simulink model "admire_linear_test_lin_cs"  (Simulink 3.00)
settings: Solver=ode4  StartTime=0.0  StopTime=30  FixedStep=0.008  RelTol=1e-3
undefined symbols (not defined in the file or in its folder): Abare, Afcs_cs, Bbare, Bfcs_cs, Cbare, Cfcs_cs, Dbare, ddc_bw, ddc_rate, ddei_bw, ddei_rate, ddey_bw, ddey_rate, ddle_bw, ddle_rate, ddr_bw, ddr_rate, Dfcs_cs, Mach, rlimit_c, rlimit_ie, rlimit_le, rlimit_oe, rlimit_r, y0bare
libraries: simulink_extras x16
settings Model: TimeSaveName=tout_lin  OutputSaveName=yout_lin  LastModifiedBy=hkg

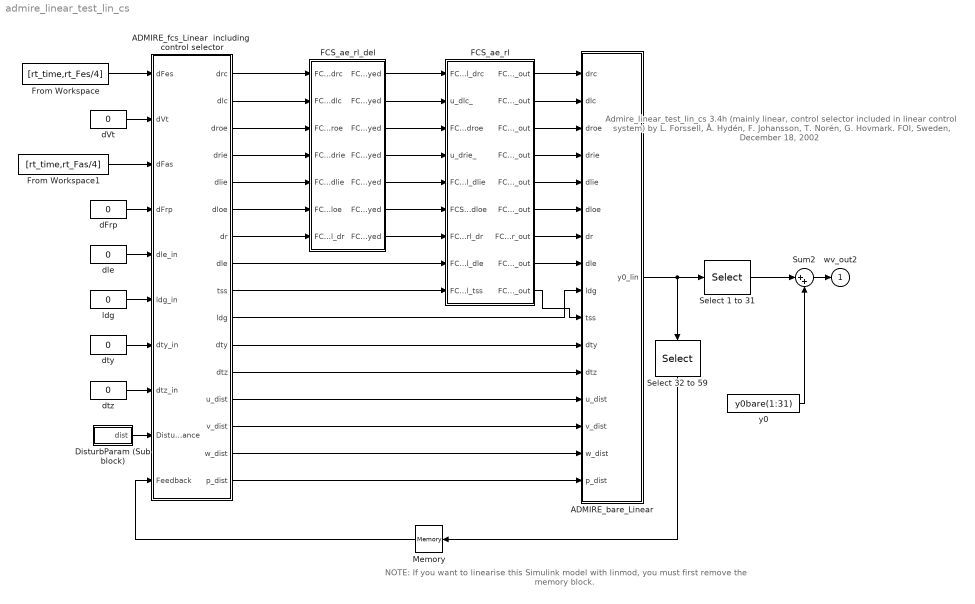
== system admire_linear_test_lin_cs ==
  note: Admire_linear_test_lin_cs 3.4h
      | (mainly linear, control selector included
      | in linear control system)
      | by  L. Forssell,
      | Å. Hydén,
      | F. Johansson,
      | T. Norén,
      | G. Hovmark.
      | FOI, Sweden,
      | December 18, 2002
  note: NOTE: If you want to linearise this Simulink model
      | with linmod, you must first
      | remove the memory block.
  ADMIRE_bare_Linear : Subsystem
  ADMIRE_fcs_Linear  including  control selector : Subsystem
  DisturbParam (Sub block) : Subsystem
  FCS_ae_rl : Subsystem
      mask Display: disp('Saturators,\nRatelimiters\nand\nActuators\n\nMach No and\nrate limiter\ndata are\ntaken from\nWorkspace\n\nAll inital\nstates empty')
  FCS_ae_rl_del : Subsystem
      mask Display: disp('Total\nComputer\nDelay\n\nAll inital\nstates empty')
  From Workspace : FromWorkspace  VariableName=[rt_time,rt_Fes/4]  SampleTime=0  HoldFinalValue=off
  From Workspace1 : FromWorkspace  VariableName=[rt_time,rt_Fas/4]  SampleTime=0  HoldFinalValue=off
  Memory : Memory  Orientation=left  X0=0  InheritSampleTime=off
  Select 1 to 31 : Selector  Elements=[1:31]  InputPortWidth=59
  Select 32 to 59 : Selector  Orientation=down  Elements=[32:59]  InputPortWidth=59
  Sum2 : Sum  Inputs=|++  SaturateOnIntegerOverflow=on
  dFrp : Constant  Value=0
  dVt : Constant  Value=0
  dle : Constant  Value=0
  dty : Constant  Value=0
  dtz : Constant  Value=0
  ldg : Constant  Value=0
  y0 : Constant  Value=y0bare(1:31)
  wv_out2 : Outport  Port=1  InitialOutput=0
  wires:
  ADMIRE_fcs_Linear  including  control selector/16(p_dist) -> ADMIRE_bare_Linear/16(p_dist)
  ADMIRE_fcs_Linear  including  control selector/12(dtz) -> ADMIRE_bare_Linear/12(dtz)
  ADMIRE_fcs_Linear  including  control selector/11(dty) -> ADMIRE_bare_Linear/11(dty)
  FCS_ae_rl_del/1(FCS_ae_rl_del_drc_delayed) -> FCS_ae_rl/1(FCS_ae_rl_drc)
  FCS_ae_rl_del/2(FCS_ae_rl_del_dlc_delayed) -> FCS_ae_rl/2(u_dlc_)
  FCS_ae_rl_del/3(FCS_ae_rl_del_droe_delayed) -> FCS_ae_rl/3(FCS_ae_rl_droe)
  FCS_ae_rl_del/4(FCS_ae_rl_del_drie_delayed) -> FCS_ae_rl/4(u_drie_)
  FCS_ae_rl_del/5(FCS_ae_rl_del_dlie_delayed) -> FCS_ae_rl/5(FCS_ae_rl_dlie)
  FCS_ae_rl_del/6(FCS_ae_rl_del_dloe_delayed) -> FCS_ae_rl/6(FCS_ae_rl_dloe)
  FCS_ae_rl_del/7(FCS_ae_rl_del_dr_delayed) -> FCS_ae_rl/7(FCS_ae_rl_dr)
  ADMIRE_fcs_Linear  including  control selector/8(dle) -> FCS_ae_rl/8(FCS_ae_rl_dle)
  ADMIRE_fcs_Linear  including  control selector/9(tss) -> FCS_ae_rl/9(FCS_ae_rl_tss)
  ADMIRE_fcs_Linear  including  control selector/10(ldg) -> ADMIRE_bare_Linear/9(ldg)
  ADMIRE_fcs_Linear  including  control selector/13(u_dist) -> ADMIRE_bare_Linear/13(u_dist)
  ADMIRE_fcs_Linear  including  control selector/14(v_dist) -> ADMIRE_bare_Linear/14(v_dist)
  ADMIRE_fcs_Linear  including  control selector/15(w_dist) -> ADMIRE_bare_Linear/15(w_dist)
  FCS_ae_rl/1(FCS_ae_rl_drc_out) -> ADMIRE_bare_Linear/1(drc)
  FCS_ae_rl/2(FCS_ae_rl_dlc_out) -> ADMIRE_bare_Linear/2(dlc)
  FCS_ae_rl/3(FCS_ae_rl_droe_out) -> ADMIRE_bare_Linear/3(droe)
  FCS_ae_rl/4(FCS_ae_rl_drie_out) -> ADMIRE_bare_Linear/4(drie)
  FCS_ae_rl/5(FCS_ae_rl_dlie_out) -> ADMIRE_bare_Linear/5(dlie)
  FCS_ae_rl/6(FCS_ae_rl_dloe_out) -> ADMIRE_bare_Linear/6(dloe)
  FCS_ae_rl/7(FCS_ae_rl_dr_out) -> ADMIRE_bare_Linear/7(dr)
  FCS_ae_rl/8(FCS_ae_rl_dle_out) -> ADMIRE_bare_Linear/8(dle)
  FCS_ae_rl/9(FCS_ae_rl_tss_out) -> ADMIRE_bare_Linear/10(tss)
  ADMIRE_bare_Linear/1(y0_lin) -> Select 1 to 31/1, Select 32 to 59/1
  Select 32 to 59/1 -> Memory/1
  Sum2/1 -> wv_out2/1
  y0/1 -> Sum2/2
  Select 1 to 31/1 -> Sum2/1
  Memory/1 -> ADMIRE_fcs_Linear  including  control selector/10(Feedback)
  ADMIRE_fcs_Linear  including  control selector/1(drc) -> FCS_ae_rl_del/1(FCS_ae_rl_del_drc)
  ADMIRE_fcs_Linear  including  control selector/2(dlc) -> FCS_ae_rl_del/2(FCS_ae_rl_del_dlc)
  ADMIRE_fcs_Linear  including  control selector/3(droe) -> FCS_ae_rl_del/3(FCS_ae_rl_del_droe)
  ADMIRE_fcs_Linear  including  control selector/4(drie) -> FCS_ae_rl_del/4(FCS_ae_rl_del_drie)
  ADMIRE_fcs_Linear  including  control selector/5(dlie) -> FCS_ae_rl_del/5(FCS_ae_rl_del_dlie)
  ADMIRE_fcs_Linear  including  control selector/6(dloe) -> FCS_ae_rl_del/6(FCS_ae_rl_del_dloe)
  ADMIRE_fcs_Linear  including  control selector/7(dr) -> FCS_ae_rl_del/7(FCS_ae_rl_del_dr)
  From Workspace/1 -> ADMIRE_fcs_Linear  including  control selector/1(dFes)
  dVt/1 -> ADMIRE_fcs_Linear  including  control selector/2(dVt)
  From Workspace1/1 -> ADMIRE_fcs_Linear  including  control selector/3(dFas)
  dFrp/1 -> ADMIRE_fcs_Linear  including  control selector/4(dFrp)
  dle/1 -> ADMIRE_fcs_Linear  including  control selector/5(dle_in)
  ldg/1 -> ADMIRE_fcs_Linear  including  control selector/6(ldg_in)
  dty/1 -> ADMIRE_fcs_Linear  including  control selector/7(dty_in)
  dtz/1 -> ADMIRE_fcs_Linear  including  control selector/8(dtz_in)
  DisturbParam (Sub block)/1(dist) -> ADMIRE_fcs_Linear  including  control selector/9(Disturbance)

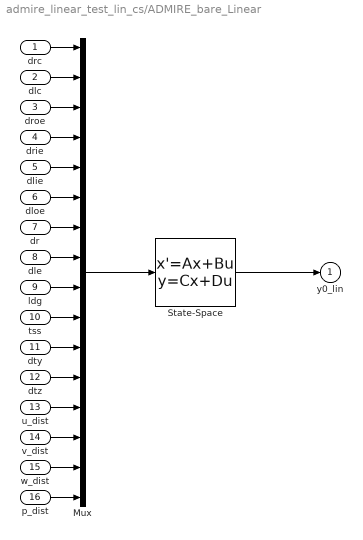
== system admire_linear_test_lin_cs/ADMIRE_bare_Linear ==
  drc : Inport  Port=1  PortWidth=-1  SampleTime=-1  DataType=auto
      settings: SignalType=auto
  dlc : Inport  Port=2  PortWidth=-1  SampleTime=-1  DataType=auto
      settings: SignalType=auto
  droe : Inport  Port=3  PortWidth=-1  SampleTime=-1  DataType=auto
      settings: SignalType=auto
  drie : Inport  Port=4  PortWidth=-1  SampleTime=-1  DataType=auto
      settings: SignalType=auto
  dlie : Inport  Port=5  PortWidth=-1  SampleTime=-1  DataType=auto
      settings: SignalType=auto
  dloe : Inport  Port=6  PortWidth=-1  SampleTime=-1  DataType=auto
      settings: SignalType=auto
  dr : Inport  Port=7  PortWidth=-1  SampleTime=-1  DataType=auto
      settings: SignalType=auto
  dle : Inport  Port=8  PortWidth=-1  SampleTime=-1  DataType=auto
      settings: SignalType=auto
  ldg : Inport  Port=9  PortWidth=-1  SampleTime=-1  DataType=auto
      settings: SignalType=auto
  tss : Inport  Port=10  PortWidth=-1  SampleTime=-1  DataType=auto
      settings: SignalType=auto
  dty : Inport  Port=11  PortWidth=-1  SampleTime=-1  DataType=auto
      settings: SignalType=auto
  dtz : Inport  Port=12  PortWidth=-1  SampleTime=-1  DataType=auto
      settings: SignalType=auto
  u_dist : Inport  Port=13  PortWidth=-1  SampleTime=-1  DataType=auto
      settings: SignalType=auto
  v_dist : Inport  Port=14  PortWidth=-1  SampleTime=-1  DataType=auto
      settings: SignalType=auto
  w_dist : Inport  Port=15  PortWidth=-1  SampleTime=-1  DataType=auto
      settings: SignalType=auto
  p_dist : Inport  Port=16  PortWidth=-1  SampleTime=-1  DataType=auto
      settings: SignalType=auto
  Mux : Mux  Inputs=16
      settings: DisplayOption=none
  State-Space : StateSpace  A=Abare  B=Bbare  C=Cbare  D=Dbare  X0=[]
  y0_lin : Outport  Port=1  InitialOutput=0
  wires:
  w_dist/1 -> Mux/15
  p_dist/1 -> Mux/16
  drc/1 -> Mux/1
  dlc/1 -> Mux/2
  droe/1 -> Mux/3
  drie/1 -> Mux/4
  dlie/1 -> Mux/5
  dloe/1 -> Mux/6
  dr/1 -> Mux/7
  dle/1 -> Mux/8
  ldg/1 -> Mux/9
  tss/1 -> Mux/10
  dty/1 -> Mux/11
  dtz/1 -> Mux/12
  u_dist/1 -> Mux/13
  v_dist/1 -> Mux/14
  Mux/1 -> State-Space/1
  State-Space/1 -> y0_lin/1

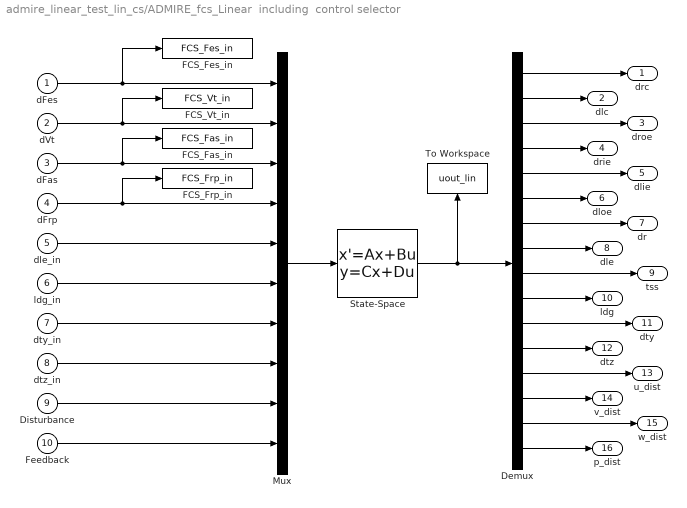
== system admire_linear_test_lin_cs/ADMIRE_fcs_Linear  including  control selector ==
  dFes : Inport  Port=1  PortWidth=-1  SampleTime=-1  DataType=auto
      settings: SignalType=auto
  dVt : Inport  Port=2  PortWidth=-1  SampleTime=-1  DataType=auto
      settings: SignalType=auto
  dFas : Inport  Port=3  PortWidth=-1  SampleTime=-1  DataType=auto
      settings: SignalType=auto
  dFrp : Inport  Port=4  PortWidth=-1  SampleTime=-1  DataType=auto
      settings: SignalType=auto
  dle_in : Inport  Port=5  PortWidth=-1  SampleTime=-1  DataType=auto
      settings: SignalType=auto
  ldg_in : Inport  Port=6  PortWidth=-1  SampleTime=-1  DataType=auto
      settings: SignalType=auto
  dty_in : Inport  Port=7  PortWidth=-1  SampleTime=-1  DataType=auto
      settings: SignalType=auto
  dtz_in : Inport  Port=8  PortWidth=-1  SampleTime=-1  DataType=auto
      settings: SignalType=auto
  Disturbance : Inport  Port=9  PortWidth=-1  SampleTime=-1  DataType=auto
      settings: SignalType=auto
  Feedback : Inport  Port=10  PortWidth=-1  SampleTime=-1  DataType=auto
      settings: SignalType=auto
  Demux : Demux  Outputs=16
  FCS_Fas_in : ToWorkspace  VariableName=FCS_Fas_in  SampleTime=-1  SaveFormat=Matrix
  FCS_Fes_in : ToWorkspace  VariableName=FCS_Fes_in  SampleTime=-1  SaveFormat=Matrix
  FCS_Frp_in : ToWorkspace  VariableName=FCS_Frp_in  SampleTime=-1  SaveFormat=Matrix
  FCS_Vt_in : ToWorkspace  VariableName=FCS_Vt_in  SampleTime=-1  SaveFormat=Matrix
  Mux : Mux  Inputs=10
  State-Space : StateSpace  A=Afcs_cs  B=Bfcs_cs  C=Cfcs_cs  D=Dfcs_cs  X0=[]
  To Workspace : ToWorkspace  VariableName=uout_lin  SampleTime=-1  SaveFormat=Matrix
      settings: Orientation=up
  drc : Outport  Port=1
  dlc : Outport  Port=2
  droe : Outport  Port=3
  drie : Outport  Port=4
  dlie : Outport  Port=5
  dloe : Outport  Port=6
  dr : Outport  Port=7
  dle : Outport  Port=8
  tss : Outport  Port=9
  ldg : Outport  Port=10
  dty : Outport  Port=11
  dtz : Outport  Port=12
  u_dist : Outport  Port=13
  v_dist : Outport  Port=14
  w_dist : Outport  Port=15
  p_dist : Outport  Port=16
  wires:
  Mux/1 -> State-Space/1
  dle_in/1 -> Mux/5
  ldg_in/1 -> Mux/6
  dty_in/1 -> Mux/7
  dtz_in/1 -> Mux/8
  Disturbance/1 -> Mux/9
  Feedback/1 -> Mux/10
  Demux/1 -> drc/1
  Demux/2 -> dlc/1
  Demux/7 -> dr/1
  Demux/8 -> dle/1
  Demux/10 -> ldg/1
  Demux/11 -> dty/1
  Demux/12 -> dtz/1
  Demux/13 -> u_dist/1
  Demux/14 -> v_dist/1
  Demux/15 -> w_dist/1
  Demux/16 -> p_dist/1
  Demux/3 -> droe/1
  Demux/4 -> drie/1
  Demux/5 -> dlie/1
  Demux/6 -> dloe/1
  Demux/9 -> tss/1
  State-Space/1 -> Demux/1, To Workspace/1
  dFes/1 -> Mux/1, FCS_Fes_in/1
  dVt/1 -> Mux/2, FCS_Vt_in/1
  dFrp/1 -> Mux/4, FCS_Frp_in/1
  dFas/1 -> Mux/3, FCS_Fas_in/1

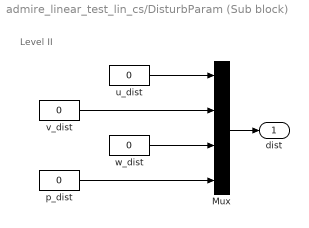
== system admire_linear_test_lin_cs/DisturbParam (Sub block) ==
  note: Level II
  Mux : Mux  Inputs=4
      settings: DisplayOption=none
  "p_dist " : Constant  Value=0
  "u_dist " : Constant  Value=0
  "v_dist " : Constant  Value=0
  "w_dist " : Constant  Value=0
  dist : Outport  Port=1
  wires:
  "p_dist "/1 -> Mux/4
  "w_dist "/1 -> Mux/3
  "v_dist "/1 -> Mux/2
  "u_dist "/1 -> Mux/1
  Mux/1 -> dist/1

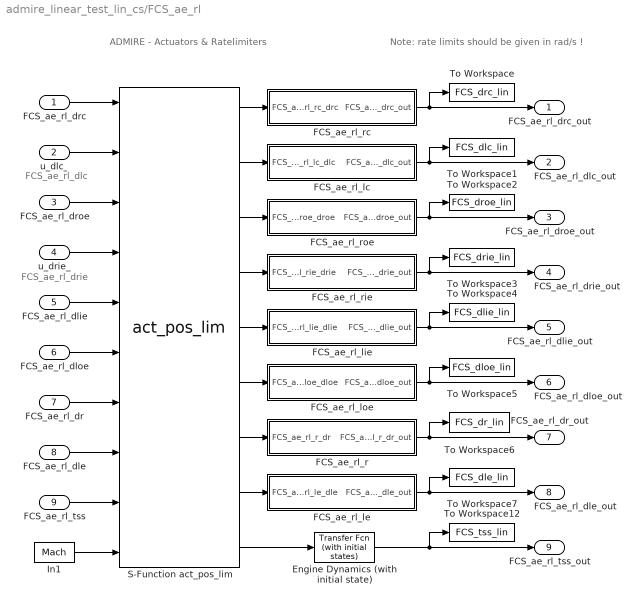
== system admire_linear_test_lin_cs/FCS_ae_rl ==
  note: Note: rate limits should be given
      | in rad/s !
  note: FCS_ae_rl_dlc
  note: FCS_ae_rl_drie
  note: ADMIRE - Actuators & Ratelimiters
  FCS_ae_rl_drc : Inport  Port=1  PortWidth=-1  SampleTime=-1  DataType=auto
      settings: SignalType=auto
  u_dlc_ : Inport  Port=2  PortWidth=-1  SampleTime=-1  DataType=auto
      settings: SignalType=auto
  FCS_ae_rl_droe : Inport  Port=3  PortWidth=-1  SampleTime=-1  DataType=auto
      settings: SignalType=auto
  u_drie_ : Inport  Port=4  PortWidth=-1  SampleTime=-1  DataType=auto
      settings: SignalType=auto
  FCS_ae_rl_dlie : Inport  Port=5  PortWidth=-1  SampleTime=-1  DataType=auto
      settings: SignalType=auto
  FCS_ae_rl_dloe : Inport  Port=6  PortWidth=-1  SampleTime=-1  DataType=auto
      settings: SignalType=auto
  FCS_ae_rl_dr : Inport  Port=7  PortWidth=-1  SampleTime=-1  DataType=auto
      settings: SignalType=auto
  FCS_ae_rl_dle : Inport  Port=8  PortWidth=-1  SampleTime=-1  DataType=auto
      settings: SignalType=auto
  FCS_ae_rl_tss : Inport  Port=9  PortWidth=-1  SampleTime=-1  DataType=auto
      settings: SignalType=auto
  Engine Dynamics (with initial state) : simulink_extras/Additional Linear/Transfer Fcn (with initial states)  N=[1]  D="[2  1]"  X0=[0]
  FCS_ae_rl_lc : Subsystem
      mask Display: disp(' Ratelimiter and Dynamics\nServo: lc')
  FCS_ae_rl_le : Subsystem
      mask Display: disp(' Ratelimiter and Dynamics\nServo: le')
  FCS_ae_rl_lie : Subsystem
      mask Display: disp(' Ratelimiter and Dynamics\nServo: lie')
  FCS_ae_rl_loe : Subsystem
      mask Display: disp(' Ratelimiter and Dynamics\nServo: loe')
  FCS_ae_rl_r : Subsystem
      mask Display: disp(' Ratelimiter and Dynamics\nServo: r')
  FCS_ae_rl_rc : Subsystem
      mask Display: disp(' Ratelimiter and Dynamics\nServo: rc')
  FCS_ae_rl_rie : Subsystem
      mask Display: disp(' Ratelimiter and Dynamics\nServo: rie')
  FCS_ae_rl_roe : Subsystem
      mask Display: disp(' Ratelimiter and Dynamics\nServo: roe')
  In1 : Constant  Value=Mach
  S-Function act_pos_lim : S-Function  FunctionName=act_pos_lim  PortCounts=[]  SFunctionModules=''
      mask Display:
      | plot([-30 30],[-30 30])
      | plot([0 0],[-30 30])
      | plot([-50 50],[0 0])
      | plot([30 50],[30 30])
      | plot([-50 -30],[-30 -30])
      | plot([-5 0],[25 30])
      | plot([5 0],[25 30])
      | plot([45 50],[3 0])
      | plot([45 50],[-3 0])
      | text(-21,26,'out')
      | text(30,-2,'in')
  To Workspace : ToWorkspace  VariableName=FCS_drc_lin  SampleTime=-1  SaveFormat=Matrix
  To Workspace1 : ToWorkspace  VariableName=FCS_dlc_lin  SampleTime=-1  SaveFormat=Matrix
  To Workspace12 : ToWorkspace  VariableName=FCS_tss_lin  SampleTime=-1  SaveFormat=Matrix
  To Workspace2 : ToWorkspace  VariableName=FCS_droe_lin  SampleTime=-1  SaveFormat=Matrix
  To Workspace3 : ToWorkspace  VariableName=FCS_drie_lin  SampleTime=-1  SaveFormat=Matrix
  To Workspace4 : ToWorkspace  VariableName=FCS_dlie_lin  SampleTime=-1  SaveFormat=Matrix
  To Workspace5 : ToWorkspace  VariableName=FCS_dloe_lin  SampleTime=-1  SaveFormat=Matrix
  To Workspace6 : ToWorkspace  VariableName=FCS_dr_lin  SampleTime=-1  SaveFormat=Matrix
  To Workspace7 : ToWorkspace  VariableName=FCS_dle_lin  SampleTime=-1  SaveFormat=Matrix
  FCS_ae_rl_drc_out : Outport  Port=1
  FCS_ae_rl_dlc_out : Outport  Port=2
  FCS_ae_rl_droe_out : Outport  Port=3
  FCS_ae_rl_drie_out : Outport  Port=4
  FCS_ae_rl_dlie_out : Outport  Port=5
  FCS_ae_rl_dloe_out : Outport  Port=6
  FCS_ae_rl_dr_out : Outport  Port=7
  FCS_ae_rl_dle_out : Outport  Port=8
  FCS_ae_rl_tss_out : Outport  Port=9
  wires:
  S-Function act_pos_lim/2 -> FCS_ae_rl_lc/1(FCS_ae_rl_lc_dlc)
  S-Function act_pos_lim/3 -> FCS_ae_rl_roe/1(FCS_ae_rl_roe_droe)
  S-Function act_pos_lim/5 -> FCS_ae_rl_lie/1(FCS_ae_rl_lie_dlie)
  S-Function act_pos_lim/6 -> FCS_ae_rl_loe/1(FCS_ae_rl_loe_dloe)
  S-Function act_pos_lim/7 -> FCS_ae_rl_r/1(FCS_ae_rl_r_dr)
  S-Function act_pos_lim/8 -> FCS_ae_rl_le/1(FCS_ae_rl_le_dle)
  S-Function act_pos_lim/9 -> Engine Dynamics (with initial state)/1
  S-Function act_pos_lim/1 -> FCS_ae_rl_rc/1(FCS_ae_rl_rc_drc)
  S-Function act_pos_lim/4 -> FCS_ae_rl_rie/1(FCS_ae_rl_rie_drie)
  In1/1 -> S-Function act_pos_lim/10
  u_dlc_/1 -> S-Function act_pos_lim/2
  FCS_ae_rl_drc/1 -> S-Function act_pos_lim/1
  FCS_ae_rl_droe/1 -> S-Function act_pos_lim/3
  FCS_ae_rl_dlie/1 -> S-Function act_pos_lim/5
  FCS_ae_rl_dloe/1 -> S-Function act_pos_lim/6
  FCS_ae_rl_dr/1 -> S-Function act_pos_lim/7
  u_drie_/1 -> S-Function act_pos_lim/4
  FCS_ae_rl_dle/1 -> S-Function act_pos_lim/8
  FCS_ae_rl_tss/1 -> S-Function act_pos_lim/9
  FCS_ae_rl_rc/1(FCS_ae_rl_rc_drc_out) -> To Workspace/1, FCS_ae_rl_drc_out/1
  FCS_ae_rl_lc/1(FCS_ae_rl_lc_dlc_out) -> To Workspace1/1, FCS_ae_rl_dlc_out/1
  Engine Dynamics (with initial state)/1 -> To Workspace12/1, FCS_ae_rl_tss_out/1
  FCS_ae_rl_le/1(FCS_ae_rl_le_dle_out) -> To Workspace7/1, FCS_ae_rl_dle_out/1
  FCS_ae_rl_r/1(FCS_ae_rl_r_dr_out) -> To Workspace6/1, FCS_ae_rl_dr_out/1
  FCS_ae_rl_loe/1(FCS_ae_rl_loe_dloe_out) -> To Workspace5/1, FCS_ae_rl_dloe_out/1
  FCS_ae_rl_lie/1(FCS_ae_rl_lie_dlie_out) -> To Workspace4/1, FCS_ae_rl_dlie_out/1
  FCS_ae_rl_roe/1(FCS_ae_rl_roe_droe_out) -> To Workspace2/1, FCS_ae_rl_droe_out/1
  FCS_ae_rl_rie/1(FCS_ae_rl_rie_drie_out) -> To Workspace3/1, FCS_ae_rl_drie_out/1

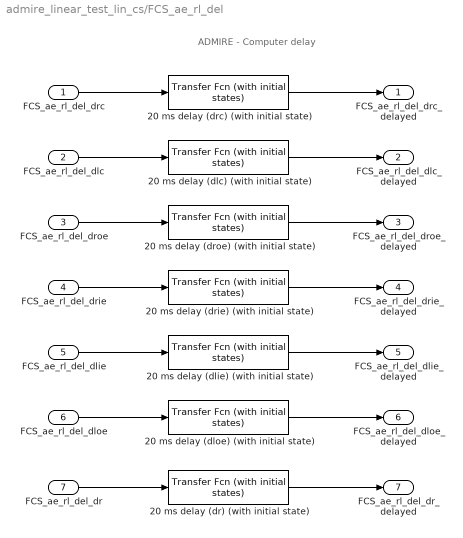
== system admire_linear_test_lin_cs/FCS_ae_rl_del ==
  note: ADMIRE - Computer delay
  FCS_ae_rl_del_drc : Inport  Port=1  PortWidth=-1  SampleTime=-1  DataType=auto
      settings: SignalType=auto
  FCS_ae_rl_del_dlc : Inport  Port=2  PortWidth=-1  SampleTime=-1  DataType=auto
      settings: SignalType=auto
  FCS_ae_rl_del_droe : Inport  Port=3  PortWidth=-1  SampleTime=-1  DataType=auto
      settings: SignalType=auto
  FCS_ae_rl_del_drie : Inport  Port=4  PortWidth=-1  SampleTime=-1  DataType=auto
      settings: SignalType=auto
  FCS_ae_rl_del_dlie : Inport  Port=5  PortWidth=-1  SampleTime=-1  DataType=auto
      settings: SignalType=auto
  FCS_ae_rl_del_dloe : Inport  Port=6  PortWidth=-1  SampleTime=-1  DataType=auto
      settings: SignalType=auto
  FCS_ae_rl_del_dr : Inport  Port=7  PortWidth=-1  SampleTime=-1  DataType=auto
      settings: SignalType=auto
  20 ms delay (dlc) (with initial state) : simulink_extras/Additional Linear/Transfer Fcn (with initial states)  N=[0.000033 -0.01 1]  D=[0.000033 0.01 1]  X0=[]
  20 ms delay (dlie) (with initial state) : simulink_extras/Additional Linear/Transfer Fcn (with initial states)  N=[0.000033 -0.01 1]  D=[0.000033 0.01 1]  X0=[]
  20 ms delay (dloe) (with initial state) : simulink_extras/Additional Linear/Transfer Fcn (with initial states)  N=[0.000033 -0.01 1]  D=[0.000033 0.01 1]  X0=[]
  20 ms delay (dr) (with initial state) : simulink_extras/Additional Linear/Transfer Fcn (with initial states)  N=[0.000033 -0.01 1]  D=[0.000033 0.01 1]  X0=[]
  20 ms delay (drc) (with initial state) : simulink_extras/Additional Linear/Transfer Fcn (with initial states)  N=[0.000033 -0.01 1]  D=[0.000033 0.01 1]  X0=[]
  20 ms delay (drie) (with initial state) : simulink_extras/Additional Linear/Transfer Fcn (with initial states)  N=[0.000033 -0.01 1]  D=[0.000033 0.01 1]  X0=[]
  20 ms delay (droe) (with initial state) : simulink_extras/Additional Linear/Transfer Fcn (with initial states)  N=[0.000033 -0.01 1]  D=[0.000033 0.01 1]  X0=[]
  FCS_ae_rl_del_drc_delayed : Outport  Port=1
  FCS_ae_rl_del_dlc_delayed : Outport  Port=2
  FCS_ae_rl_del_droe_delayed : Outport  Port=3
  FCS_ae_rl_del_drie_delayed : Outport  Port=4
  FCS_ae_rl_del_dlie_delayed : Outport  Port=5
  FCS_ae_rl_del_dloe_delayed : Outport  Port=6
  FCS_ae_rl_del_dr_delayed : Outport  Port=7
  wires:
  FCS_ae_rl_del_drc/1 -> 20 ms delay (drc) (with initial state)/1
  FCS_ae_rl_del_dlc/1 -> 20 ms delay (dlc) (with initial state)/1
  FCS_ae_rl_del_droe/1 -> 20 ms delay (droe) (with initial state)/1
  FCS_ae_rl_del_drie/1 -> 20 ms delay (drie) (with initial state)/1
  FCS_ae_rl_del_dlie/1 -> 20 ms delay (dlie) (with initial state)/1
  FCS_ae_rl_del_dloe/1 -> 20 ms delay (dloe) (with initial state)/1
  FCS_ae_rl_del_dr/1 -> 20 ms delay (dr) (with initial state)/1
  20 ms delay (drc) (with initial state)/1 -> FCS_ae_rl_del_drc_delayed/1
  20 ms delay (dlc) (with initial state)/1 -> FCS_ae_rl_del_dlc_delayed/1
  20 ms delay (droe) (with initial state)/1 -> FCS_ae_rl_del_droe_delayed/1
  20 ms delay (drie) (with initial state)/1 -> FCS_ae_rl_del_drie_delayed/1
  20 ms delay (dlie) (with initial state)/1 -> FCS_ae_rl_del_dlie_delayed/1
  20 ms delay (dloe) (with initial state)/1 -> FCS_ae_rl_del_dloe_delayed/1
  20 ms delay (dr) (with initial state)/1 -> FCS_ae_rl_del_dr_delayed/1

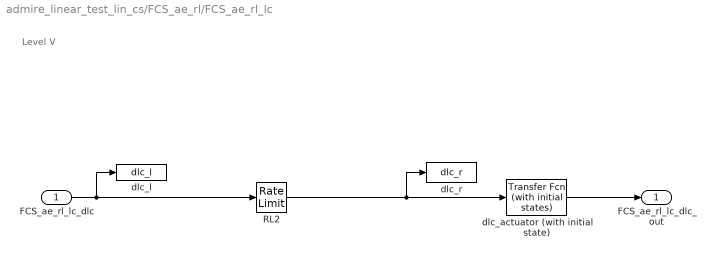
== system admire_linear_test_lin_cs/FCS_ae_rl/FCS_ae_rl_lc ==
  note: Level V
  FCS_ae_rl_lc_dlc : Inport  Port=1  PortWidth=-1  SampleTime=-1  DataType=auto
      settings: SignalType=auto
  RL2 : RateLimiter  RisingSlewLimit=rlimit_c+ddc_rate  FallingSlewLimit=-rlimit_c-ddc_rate
  dlc_actuator (with initial state) : simulink_extras/Additional Linear/Transfer Fcn (with initial states)  N=[1]  D="[0.05+ddc_bw  1]"  X0=[]
  dlc_l : ToWorkspace  VariableName=dlc_l  SampleTime=0  SaveFormat=Matrix
      settings: Buffer=10000
  dlc_r : ToWorkspace  VariableName=dlc_r  SampleTime=0  SaveFormat=Matrix
      settings: Buffer=10000
  FCS_ae_rl_lc_dlc_out : Outport  Port=1  InitialOutput=0
  wires:
  FCS_ae_rl_lc_dlc/1 -> dlc_l/1, RL2/1
  dlc_actuator (with initial state)/1 -> FCS_ae_rl_lc_dlc_out/1
  RL2/1 -> dlc_r/1, dlc_actuator (with initial state)/1

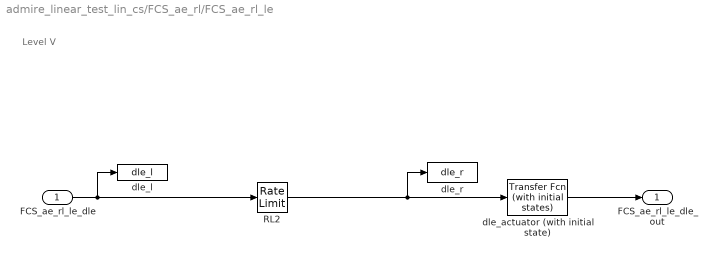
== system admire_linear_test_lin_cs/FCS_ae_rl/FCS_ae_rl_le ==
  note: Level V
  FCS_ae_rl_le_dle : Inport  Port=1  PortWidth=-1  SampleTime=-1  DataType=auto
      settings: SignalType=auto
  RL2 : RateLimiter  RisingSlewLimit=rlimit_le+ddle_rate  FallingSlewLimit=-rlimit_le-ddle_rate
  dle_actuator (with initial state) : simulink_extras/Additional Linear/Transfer Fcn (with initial states)  N=[1]  D="[0.05+ddle_bw  1]"  X0=[0]
  dle_l : ToWorkspace  VariableName=dle_l  SampleTime=0  SaveFormat=Matrix
      settings: Buffer=10000
  dle_r : ToWorkspace  VariableName=dle_r  SampleTime=0  SaveFormat=Matrix
      settings: Buffer=10000
  FCS_ae_rl_le_dle_out : Outport  Port=1  InitialOutput=0
  wires:
  FCS_ae_rl_le_dle/1 -> dle_l/1, RL2/1
  dle_actuator (with initial state)/1 -> FCS_ae_rl_le_dle_out/1
  RL2/1 -> dle_r/1, dle_actuator (with initial state)/1

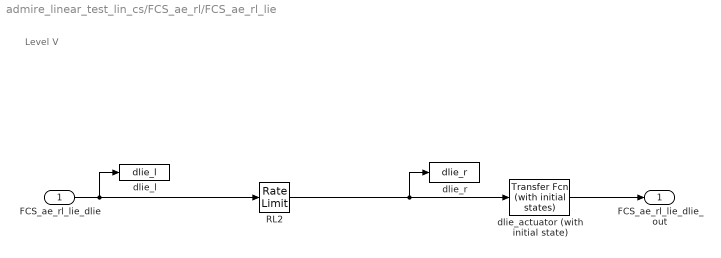
== system admire_linear_test_lin_cs/FCS_ae_rl/FCS_ae_rl_lie ==
  note: Level V
  FCS_ae_rl_lie_dlie : Inport  Port=1  PortWidth=-1  SampleTime=-1  DataType=auto
      settings: SignalType=auto
  RL2 : RateLimiter  RisingSlewLimit=rlimit_ie+ddei_rate  FallingSlewLimit=-rlimit_ie-ddei_rate
  dlie_actuator (with initial state) : simulink_extras/Additional Linear/Transfer Fcn (with initial states)  N=[1]  D="[0.05+ddei_bw  1]"  X0=[0]
  dlie_l : ToWorkspace  VariableName=dlie_l  SampleTime=0  SaveFormat=Matrix
      settings: Buffer=10000
  dlie_r : ToWorkspace  VariableName=dlie_r  SampleTime=0  SaveFormat=Matrix
      settings: Buffer=10000
  FCS_ae_rl_lie_dlie_out : Outport  Port=1  InitialOutput=0
  wires:
  dlie_actuator (with initial state)/1 -> FCS_ae_rl_lie_dlie_out/1
  FCS_ae_rl_lie_dlie/1 -> dlie_l/1, RL2/1
  RL2/1 -> dlie_actuator (with initial state)/1, dlie_r/1

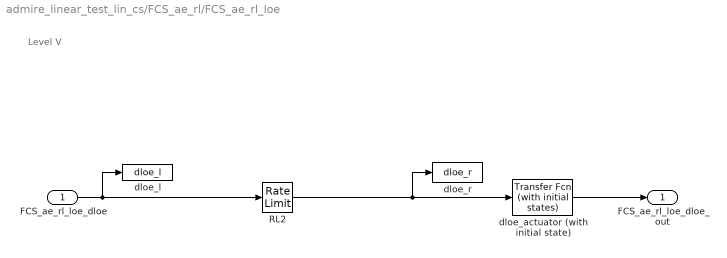
== system admire_linear_test_lin_cs/FCS_ae_rl/FCS_ae_rl_loe ==
  note: Level V
  FCS_ae_rl_loe_dloe : Inport  Port=1  PortWidth=-1  SampleTime=-1  DataType=auto
      settings: SignalType=auto
  RL2 : RateLimiter  RisingSlewLimit=rlimit_oe+ddey_rate  FallingSlewLimit=-rlimit_oe-ddey_rate
  dloe_actuator (with initial state) : simulink_extras/Additional Linear/Transfer Fcn (with initial states)  N=[1]  D="[0.05+ddey_bw  1]"  X0=[0]
  dloe_l : ToWorkspace  VariableName=dloe_l  SampleTime=0  SaveFormat=Matrix
      settings: Buffer=10000
  dloe_r : ToWorkspace  VariableName=dloe_r  SampleTime=0  SaveFormat=Matrix
      settings: Buffer=10000
  FCS_ae_rl_loe_dloe_out : Outport  Port=1  InitialOutput=0
  wires:
  FCS_ae_rl_loe_dloe/1 -> dloe_l/1, RL2/1
  dloe_actuator (with initial state)/1 -> FCS_ae_rl_loe_dloe_out/1
  RL2/1 -> dloe_r/1, dloe_actuator (with initial state)/1

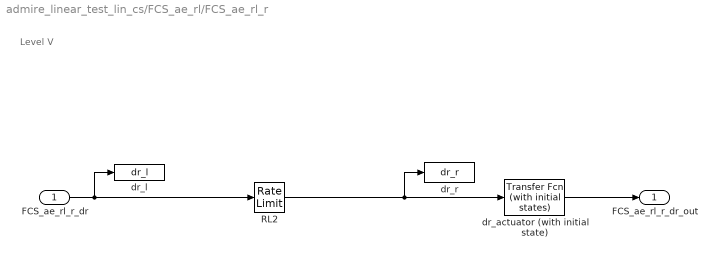
== system admire_linear_test_lin_cs/FCS_ae_rl/FCS_ae_rl_r ==
  note: Level V
  FCS_ae_rl_r_dr : Inport  Port=1  PortWidth=-1  SampleTime=-1  DataType=auto
      settings: SignalType=auto
  RL2 : RateLimiter  RisingSlewLimit=rlimit_r+ddr_rate  FallingSlewLimit=-rlimit_r-ddr_rate
  dr_actuator (with initial state) : simulink_extras/Additional Linear/Transfer Fcn (with initial states)  N=[1]  D="[0.05+ddr_bw  1]"  X0=[0]
  dr_l : ToWorkspace  VariableName=dr_l  SampleTime=0  SaveFormat=Matrix
      settings: Buffer=10000
  dr_r : ToWorkspace  VariableName=dr_r  SampleTime=0  SaveFormat=Matrix
      settings: Buffer=10000
  FCS_ae_rl_r_dr_out : Outport  Port=1  InitialOutput=0
  wires:
  dr_actuator (with initial state)/1 -> FCS_ae_rl_r_dr_out/1
  FCS_ae_rl_r_dr/1 -> dr_l/1, RL2/1
  RL2/1 -> dr_actuator (with initial state)/1, dr_r/1

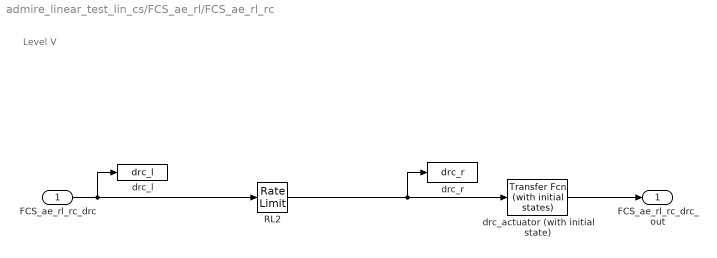
== system admire_linear_test_lin_cs/FCS_ae_rl/FCS_ae_rl_rc ==
  note: Level V
  FCS_ae_rl_rc_drc : Inport  Port=1  PortWidth=-1  SampleTime=-1  DataType=auto
      settings: SignalType=auto
  RL2 : RateLimiter  RisingSlewLimit=rlimit_c+ddc_rate  FallingSlewLimit=-rlimit_c-ddc_rate
  drc_actuator (with initial state) : simulink_extras/Additional Linear/Transfer Fcn (with initial states)  N=[1]  D="[0.05+ddc_bw  1]"  X0=[]
  drc_l : ToWorkspace  VariableName=drc_l  SampleTime=0  SaveFormat=Matrix
      settings: Buffer=10000
  drc_r : ToWorkspace  VariableName=drc_r  SampleTime=0  SaveFormat=Matrix
      settings: Buffer=10000
  FCS_ae_rl_rc_drc_out : Outport  Port=1  InitialOutput=0
  wires:
  drc_actuator (with initial state)/1 -> FCS_ae_rl_rc_drc_out/1
  FCS_ae_rl_rc_drc/1 -> drc_l/1, RL2/1
  RL2/1 -> drc_actuator (with initial state)/1, drc_r/1

== system admire_linear_test_lin_cs/FCS_ae_rl/FCS_ae_rl_rie ==
  note: Level V
  FCS_ae_rl_rie_drie : Inport  Port=1  PortWidth=-1  SampleTime=-1  DataType=auto
      settings: SignalType=auto
  RL2 : RateLimiter  RisingSlewLimit=rlimit_ie+ddei_rate  FallingSlewLimit=-rlimit_ie-ddei_rate
  drie_actuator (with initial state) : simulink_extras/Additional Linear/Transfer Fcn (with initial states)  N=[1]  D="[0.05+ddei_bw  1]"  X0=[]
  drie_l : ToWorkspace  VariableName=drie_l  SampleTime=0  SaveFormat=Matrix
      settings: Buffer=10000
  drie_r : ToWorkspace  VariableName=drie_r  SampleTime=0  SaveFormat=Matrix
      settings: Buffer=10000
  FCS_ae_rl_rie_drie_out : Outport  Port=1  InitialOutput=0
  wires:
  FCS_ae_rl_rie_drie/1 -> drie_l/1, RL2/1
  drie_actuator (with initial state)/1 -> FCS_ae_rl_rie_drie_out/1
  RL2/1 -> drie_r/1, drie_actuator (with initial state)/1

== system admire_linear_test_lin_cs/FCS_ae_rl/FCS_ae_rl_roe ==
  note: Level V
  FCS_ae_rl_roe_droe : Inport  Port=1  PortWidth=-1  SampleTime=-1  DataType=auto
      settings: SignalType=auto
  RL2 : RateLimiter  RisingSlewLimit=rlimit_oe+ddey_rate  FallingSlewLimit=-rlimit_oe-ddey_rate
  droe_actuator (with initial state) : simulink_extras/Additional Linear/Transfer Fcn (with initial states)  N=[1]  D="[0.05+ddey_bw  1]"  X0=[]
  droe_l : ToWorkspace  VariableName=droe_l  SampleTime=0  SaveFormat=Matrix
      settings: Buffer=10000
  droe_r : ToWorkspace  VariableName=droe_r  SampleTime=0  SaveFormat=Matrix
      settings: Buffer=10000
  FCS_ae_rl_roe_droe_out : Outport  Port=1  InitialOutput=0
  wires:
  droe_actuator (with initial state)/1 -> FCS_ae_rl_roe_droe_out/1
  FCS_ae_rl_roe_droe/1 -> droe_l/1, RL2/1
  RL2/1 -> droe_actuator (with initial state)/1, droe_r/1
